simulink model "AA"  (R2020a)
settings: Solver=VariableStepAuto  StartTime=0.0  StopTime=100  RelTol=1e-3
InitFcn:
  | variableCalc
values from neighbouring files (symbols this model uses):
  Alin = [(-1).*F.*M.^(-1),0,0,0;1,0,0,0;(-1).*F.*l.^(-1).*M.^(-1),0,0,g.*l.^(-1)    ;0,0,1,0]    [Matrix.m]
  Blin = [M.^(-1);0;l.^(-1).*M.^(-1);0]    [Matrix.m]
  Clin = [0,1,0,0;0,0,0,1]    [Matrix.m]
  Gamma = [(-1),(-1).*M.*wD2.^2,F.*wD2]    [Matrix.m]
  K = [(-1/2).*g.^(-1).*((-2).*F.*g+3.*l.*lam.^3.*M),(1/4).*g.^(-1).*l.*    lam.^4.*M,(3/2).*g.^(-1).*(2.*g.*l.*lam.*M+l.^2.*lam.^3.*M),(-1/4).*g.^(    -1).*(4.*g.^2.*M+13.*g.*l.*lam.^2.*M+l.^2.*lam.^4.*M)]    [Matrix.m]
  PiMat = [0,0,wD2;0,1,0;0,0,wD2.^3.*(g+l.*wD2.^2).^(-1);0,wD2.^2.*(g+l.*wD2.^2)    .^(-1),0]    [Matrix.m]
  S = [0 0 0 ... (first row only)    [variableCalc.m]
settings Model: Creator=astolfi  LastModifiedBy=alfystar

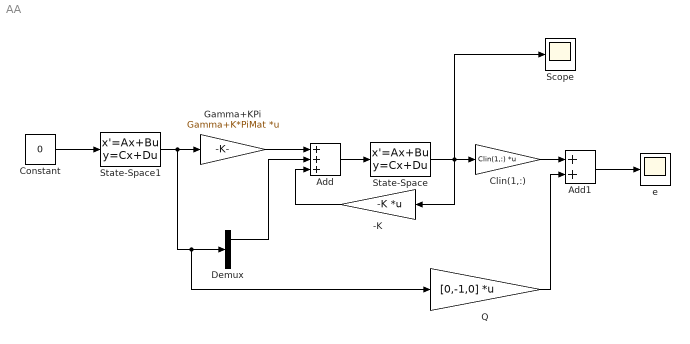
== system AA ==
  -K : Gain  Gain=-K  Multiplication=Matrix(K*u) (u vector)
  Add : Sum  Inputs=+++
  Add1 : Sum
  Clin(1,:) : Gain  Gain=Clin(1,:)  Multiplication=Matrix(K*u) (u vector)
  Constant : Constant  Value=0
  Demux : Demux  Outputs=3
  Gamma+KPi : Gain  Gain=Gamma+K*PiMat  Multiplication=Matrix(K*u) (u vector)
  Q : Gain  Gain=[0,-1,0]  Multiplication=Matrix(K*u) (u vector)
  Scope : Scope
  State-Space : StateSpace  A=Alin  B=Blin  C=eye(4)  D=zeros(4,1)  InitialCondition=rand(4,1)
  State-Space1 : StateSpace  A=S  B=[0;0;0]  C=eye(3)  D=[0;0;0]  InitialCondition=rand(1,3)
  e : Scope
  wires:
  Add/1 -> State-Space/1
  State-Space1/1 -> Q/1, Demux/1, Gamma+KPi/1
  State-Space/1 -> -K/1, Scope/1, Clin(1,:)/1
  -K/1 -> Add/3
  Gamma+KPi/1 -> Add/1
  Demux/1 -> Add/2
  Clin(1,:)/1 -> Add1/1
  Q/1 -> Add1/2
  Add1/1 -> e/1
  Constant/1 -> State-Space1/1
